simulink model "Lab1_mdl_diskr_observer"  (R2013b)
settings: Solver=ode3  StartTime=0.0  StopTime=100.0  FixedStep=10e-3  RelTol=1e-3
values from neighbouring files (symbols this model uses):
  Adk = Ad - Bd*K    [Lab1.m]
  K = place(Ad,Bd,Rp)    [Lab1.m]
  L = place(Ad',Cd',Ro)    [Lab1.m]
undefined symbols (not defined in the file or in its folder): Ad, Bd, Cd, Dd
settings Model: Creator=user  LastModifiedBy=user
settings DataIOCC: LimitDataPoints=off

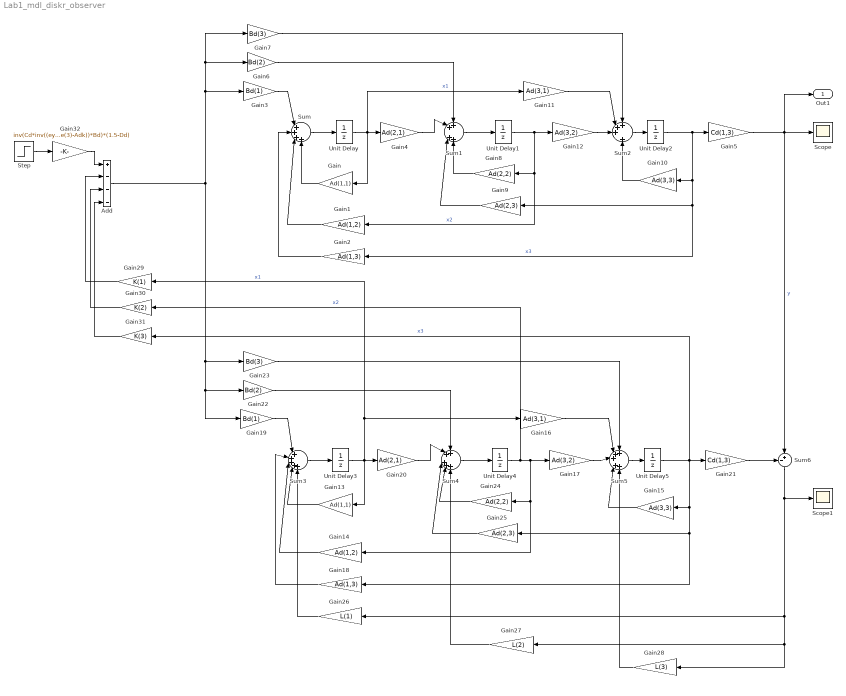
== system Lab1_mdl_diskr_observer ==
  Add : Sum  Inputs=+---
  Gain : Gain  Gain=Ad(1,1)
  Gain1 : Gain  Gain=Ad(1,2)
  Gain10 : Gain  Gain=Ad(3,3)
  Gain11 : Gain  Gain=Ad(3,1)
  Gain12 : Gain  Gain=Ad(3,2)
  Gain13 : Gain  Gain=Ad(1,1)
  Gain14 : Gain  Gain=Ad(1,2)
  Gain15 : Gain  Gain=Ad(3,3)
  Gain16 : Gain  Gain=Ad(3,1)
  Gain17 : Gain  Gain=Ad(3,2)
  Gain18 : Gain  Gain=Ad(1,3)
  Gain19 : Gain  Gain=Bd(1)
  Gain2 : Gain  Gain=Ad(1,3)
  Gain20 : Gain  Gain=Ad(2,1)
  Gain21 : Gain  Gain=Cd(1,3)
  Gain22 : Gain  Gain=Bd(2)
  Gain23 : Gain  Gain=Bd(3)
  Gain24 : Gain  Gain=Ad(2,2)
  Gain25 : Gain  Gain=Ad(2,3)
  Gain26 : Gain  Gain=L(1)
  Gain27 : Gain  Gain=L(2)
  Gain28 : Gain  Gain=L(3)
  Gain29 : Gain  Gain=K(1)
  Gain3 : Gain  Gain=Bd(1)
  Gain30 : Gain  Gain=K(2)
  Gain31 : Gain  Gain=K(3)
  Gain32 : Gain  Gain=inv(Cd*inv((eye(3)-Adk))*Bd)*(1.5-Dd)
  Gain4 : Gain  Gain=Ad(2,1)
  Gain5 : Gain  Gain=Cd(1,3)
  Gain6 : Gain  Gain=Bd(2)
  Gain7 : Gain  Gain=Bd(3)
  Gain8 : Gain  Gain=Ad(2,2)
  Gain9 : Gain  Gain=Ad(2,3)
  Scope : Scope
      settings: SaveName=Observer
  Scope1 : Scope
      settings: SaveName=Observer1
  Step : Step  Time=0  SampleTime=0.4  mask(DiscretizedSource){}
      mask init:
      | %zoh
  Sum : Sum  Inputs=|++++
  Sum1 : Sum  Inputs=++|++
  Sum2 : Sum  Inputs=+++|+
  Sum3 : Sum  Inputs=|+++++
  Sum4 : Sum  Inputs=++|+++
  Sum5 : Sum  Inputs=+++|++
  Sum6 : Sum  Inputs=-+|
  Unit Delay{,1..2,4..5} (5 alike) : UnitDelay  SampleTime=0.4
  Unit Delay3 : UnitDelay  InitialCondition=0.01  SampleTime=0.4
  Out1 : Outport
  wires:
  Unit Delay/1 -> Gain4/1, Gain11/1, Gain/1  "x1"
  Sum/1 -> Unit Delay/1
  Gain/1 -> Sum/4
  Gain1/1 -> Sum/3
  Gain2/1 -> Sum/2
  Gain3/1 -> Sum/1
  Step/1 -> Gain32/1
  Gain5/1 -> Scope/1, Out1/1, Sum6/2  "y"
  Gain4/1 -> Sum1/2
  Sum1/1 -> Unit Delay1/1
  Gain6/1 -> Sum1/1
  Sum2/1 -> Unit Delay2/1
  Gain7/1 -> Sum2/1
  Unit Delay1/1 -> Gain12/1, Gain1/1, Gain8/1  "x2"
  Gain8/1 -> Sum1/4
  Gain9/1 -> Sum1/3
  Unit Delay2/1 -> Gain5/1, Gain2/1, Gain9/1, Gain10/1  "x3"
  Gain12/1 -> Sum2/3
  Gain10/1 -> Sum2/4
  Gain11/1 -> Sum2/2
  Unit Delay3/1 -> Gain20/1, Gain29/1, Gain16/1, Gain13/1  "x1"
  Sum3/1 -> Unit Delay3/1
  Gain13/1 -> Sum3/4
  Gain14/1 -> Sum3/3
  Gain18/1 -> Sum3/2
  Gain19/1 -> Sum3/1
  Add/1 -> Gain3/1, Gain6/1, Gain7/1, Gain23/1, Gain22/1, Gain19/1
  Gain20/1 -> Sum4/2
  Sum4/1 -> Unit Delay4/1
  Gain22/1 -> Sum4/1
  Sum5/1 -> Unit Delay5/1
  Gain23/1 -> Sum5/1
  Unit Delay4/1 -> Gain14/1, Gain24/1, Gain17/1, Gain30/1  "x2"
  Gain24/1 -> Sum4/4
  Gain25/1 -> Sum4/3
  Unit Delay5/1 -> Gain18/1, Gain25/1, Gain15/1, Gain31/1, Gain21/1  "x3"
  Gain17/1 -> Sum5/3
  Gain15/1 -> Sum5/4
  Gain16/1 -> Sum5/2
  Gain21/1 -> Sum6/1
  Gain26/1 -> Sum3/5
  Sum6/1 -> Scope1/1, Gain28/1, Gain27/1, Gain26/1
  Gain27/1 -> Sum4/5
  Gain31/1 -> Add/4
  Gain30/1 -> Add/3
  Gain29/1 -> Add/2
  Gain32/1 -> Add/1
  Gain28/1 -> Sum5/5
